simulink model "zad_08_base"  (R2022b)
settings: Solver=VariableStepAuto  StartTime=0.0  StopTime=1000  RelTol=1e-3
undefined symbols (not defined in the file or in its folder): den0, num0
settings Model: Creator=mrxmi  LastModifiedBy=mrxmi

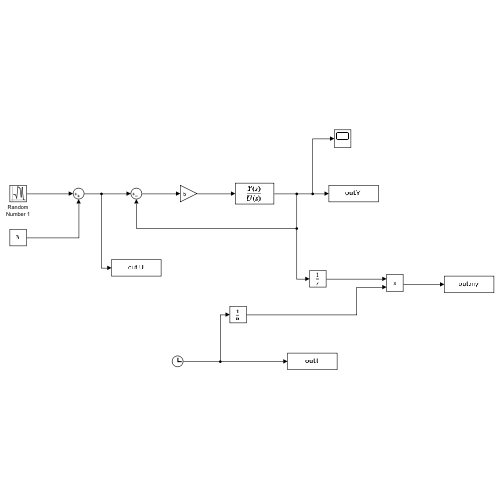
[thumbnail: Simulink's stored preview of the top-level diagram]
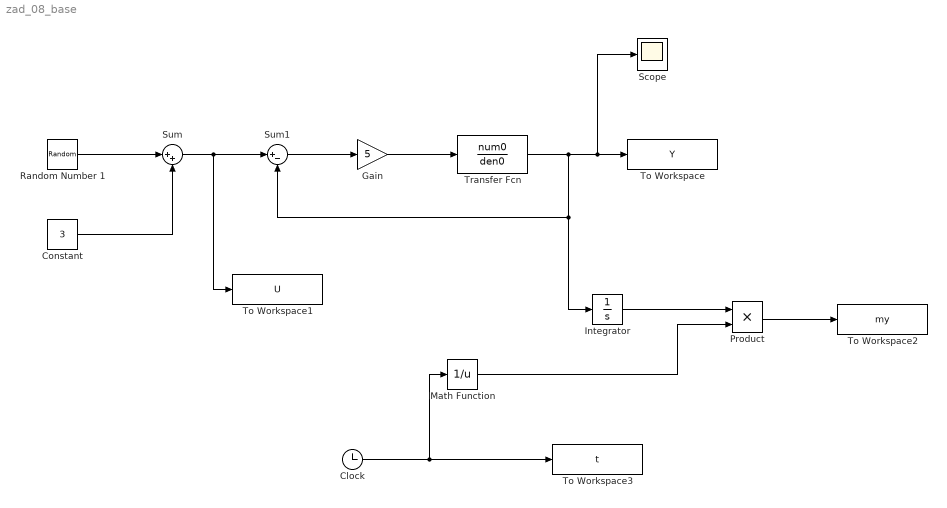
== system zad_08_base ==
  Clock : Clock
  Constant : Constant  Value=3
  Gain : Gain  Gain=5
  Integrator : Integrator
  Math Function : Math  Operator=reciprocal  SignedPower=on  RndMeth=Zero
  Product : Product
  Random Number 1 : RandomNumber  SampleTime=0.1
  Scope : Scope
  Sum : Sum  Inputs=|++
  Sum1 : Sum  Inputs=|+-
  To Workspace : ToWorkspace  VariableName=Y  SampleTime=-1
  To Workspace1 : ToWorkspace  VariableName=U  SampleTime=-1
  To Workspace2 : ToWorkspace  VariableName=my  SampleTime=-1
  To Workspace3 : ToWorkspace  VariableName=t  SampleTime=-1
  Transfer Fcn : TransferFcn  Numerator=num0  Denominator=den0
  wires:
  Random Number 1/1 -> Sum/1
  Constant/1 -> Sum/2
  Sum/1 -> To Workspace1/1, Sum1/1
  Product/1 -> To Workspace2/1
  Integrator/1 -> Product/1
  Transfer Fcn/1 -> Scope/1, To Workspace/1, Sum1/2, Integrator/1
  Gain/1 -> Transfer Fcn/1
  Sum1/1 -> Gain/1
  Math Function/1 -> Product/2
  Clock/1 -> Math Function/1, To Workspace3/1
